simulink library "Kitchen_Lib"  (R2023a)
settings: Solver=VariableStepAuto  StartTime=0.0  StopTime=10.0  RelTol=1e-3  EnableMultiTasking=on
undefined symbols (not defined in the file): Kitc_BusTyp_P, Kitc_BusTypSkyr_C, Kitc_ColrLedColrls_C, Kitc_ColrLedGrn_C, Kitc_ColrLedRed_C, Kitc_ColrLedYlw_C, Kitc_StDgnWtrTank_C, Kitc_StElecPlugScktOffByClmp50_P, Kitc_StsDlyBlink_C, Kitc_StsErrBlink_C, Kitc_StsFctAcvn_P, Kitc_StsInfoBlink_C, Kitc_StsKitchnOffAutoIgOff_P, Kitc_StsKitchnOffBySwt_P, Kitc_StsKitchnOffDoorLockd_P, Kitc_StsKitchnOffIgOff_P, Kitc_StsKitchnOffUv_P, Kitc_StsKitchnOnBySwt_P, Kitc_StsKitchnOnNVM_P, Kitc_StsLedOff_C, Kitc_StsLedOn_C, Kitc_StsLrgCnsAcv_P, Kitc_StTrfrAnSwtInstd_P, Kitc_StTrfrSwtInstd_P, Kitc_TiKitcRefgtrOffDly_P, Kitc_ULowrThdBat_C, Kitc_UUpprThdBat_C, Kitc_ValFalse_C, Kitc_ValPwmFreq2_C, Kitc_ValPwmFreq_C, Kitc_ValTrue_C
libraries: MAN_Library x50, E2E_Lib x3
(part 5 of 13)

== system Kitchen_Lib/Kitchen/100ms/Kitchn/Subsystem1/Subsystem9/BOOLEAN_TO_UINT8_Signals ==
  BOOLEAN_TO_UINT8_SignalIn : Inport
  Constant : Constant  Value=uint8(0)
  Constant1 : Constant  Value=uint8(1)
  Constant2 : Constant  Value=uint8(2)
  Constant3 : Constant  Value=uint8(3)
  Data Type Conversion : DataTypeConversion  OutDataTypeStr=uint8  SaturateOnIntegerOverflow=off  RndMeth=Floor
  Relational Operator{,1..3} (4 alike) : RelationalOperator  Operator===  OutDataTypeStr=boolean  InputSameDT=off
  SignalOff : Outport
  Signal|On : Outport  Port=2
  Error : Outport  Port=3
  NotInstalled_NotAvailable : Outport  Port=4
  wires:
  Relational Operator3/1 -> NotInstalled_NotAvailable/1
  Relational Operator2/1 -> Error/1
  Relational Operator1/1 -> Signal|On/1
  Relational Operator/1 -> SignalOff/1
  Data Type Conversion/1 -> Relational Operator/1, Relational Operator2/1, Relational Operator3/1, Relational Operator1/1
  Constant2/1 -> Relational Operator2/2
  Constant/1 -> Relational Operator/2
  BOOLEAN_TO_UINT8_SignalIn/1 -> Data Type Conversion/1
  Constant3/1 -> Relational Operator3/2
  Constant1/1 -> Relational Operator1/2

== system Kitchen_Lib/Kitchen/100ms/Kitchn/Subsystem1/Subsystem16/001_KitchnCtl/001_HostessSideButton ==
  GW_SpdGrtr3 : Inport
  DBF_StsDoor1Open : Inport  Port=2
  Kitc_StKitcHostsSideSwtUpprPart : Inport  Port=3
  Kitc_StKitcHostsSideSwtBotmPart : Inport  Port=4
  "GW_ModeExbn " : Inport  Port=5
  "GW_StUvTopPrio " : Inport  Port=6
  Kitchn_On : Inport  Port=7
  001_HostessSideTopButton : Subsystem
  002_HostessSideBottomButton : Subsystem
  Logical Operator18 : Logic  AllPortsSameDT=off  OutDataTypeStr=boolean
  Logical Operator19 : Logic  Operator=NOT  Inputs=4  AllPortsSameDT=off  OutDataTypeStr=boolean
  HostsSideTopBtnErr : Outport
  HostsSideBotmBtnErr : Outport  Port=2
  HostsSideTopBtn_ON : Outport  Port=3
  HostsSideBotmBtn_OFF : Outport  Port=4
  wires:
  Logical Operator18/1 -> 001_HostessSideTopButton/2(SwtLock), 002_HostessSideBottomButton/4(SwtLock)
  002_HostessSideBottomButton/1(HostessSideBottomButtonErr) -> HostsSideBotmBtnErr/1
  "GW_ModeExbn "/1 -> 001_HostessSideTopButton/3("GW_ModeExbn "), 002_HostessSideBottomButton/2("GW_ModeExbn ")
  001_HostessSideTopButton/2(HostessSideBottomButton_ON) -> HostsSideTopBtn_ON/1
  GW_SpdGrtr3/1 -> Logical Operator19/1
  002_HostessSideBottomButton/2(HostessSideBottomButton_OFF) -> HostsSideBotmBtn_OFF/1
  Kitchn_On/1 -> 002_HostessSideBottomButton/1(Kitchn_On), 001_HostessSideTopButton/5(Kitchn_On)
  Logical Operator19/1 -> Logical Operator18/1
  Kitc_StKitcHostsSideSwtUpprPart/1 -> 001_HostessSideTopButton/1(Kitc_StKitcHostsSideSwtUpprPart)
  001_HostessSideTopButton/1(HostessSideTopButtonErr) -> HostsSideTopBtnErr/1
  DBF_StsDoor1Open/1 -> Logical Operator18/2
  "GW_StUvTopPrio "/1 -> 001_HostessSideTopButton/4("GW_StUvTopPrio ")
  Kitc_StKitcHostsSideSwtBotmPart/1 -> 002_HostessSideBottomButton/3(Kitc_StKitcHostsSideSwtBotmPart)

== system Kitchen_Lib/Kitchen/100ms/Kitchn/Subsystem1/Subsystem16/001_KitchnCtl/002_FlipFlop ==
  Kitc_StsHostsCallAcv : Inport
  Kitc_StKitcSwtUpprPart : Inport  Port=2
  HostsSideTopBtn_ON : Inport  Port=3
  HostsSideBotmBtn_OFF : Inport  Port=4
  Kitc_StKitcSwtBotmPart : Inport  Port=5
  CLS_StDoorLockdOutd : Inport  Port=6
  "GW_StStrtNew " : Inport  Port=7
  "GW_ModeExbn " : Inport  Port=8
  "GW_StUvTopPrio " : Inport  Port=9
  GW_StClmp15 : Inport  Port=10
  ABat_StAddlBatInstd : Inport  Port=11
  GW_StEngRung : Inport  Port=12
  "GW_Ubat " : Inport  Port=13
  "GW_StClmp50Off3Sec " : Inport  Port=14
  Kitc_StDemoBd : Inport  Port=15
  Kitc_TdOff : Inport  Port=16
  KSW-KitchenControl : Subsystem
  KitchenEnable : Subsystem
  LrgCns : Outport
  Kitc_WarnLrgCns : Outport  Port=2
  Kitchn_On : Outport  Port=3
  Kitc_StsKitcAcv : Outport  Port=4
  Kitchn_HostsCallOn : Outport  Port=5
  Kitc_StLrgCns : Outport  Port=6
  Kitc_StSmlCns : Outport  Port=7
  Kitc_StWtrPump : Outport  Port=8
  Kitc_StBuzRe : Outport  Port=9
  Kitc_StKitcLi : Outport  Port=10
  Kitc_StsPwmFreq : Outport  Port=11
  wires:
  Kitc_StKitcSwtUpprPart/1 -> KitchenEnable/1(Kitc_StKitcSwtUpprPart)
  HostsSideTopBtn_ON/1 -> KitchenEnable/2(HostsSideTopBtn_ON)
  HostsSideBotmBtn_OFF/1 -> KitchenEnable/3(HostsSideBotmBtn_OFF)
  Kitc_StKitcSwtBotmPart/1 -> KitchenEnable/4(Kitc_StKitcSwtBotmPart)
  CLS_StDoorLockdOutd/1 -> [CLS_StDoorLockdOutd]
  "GW_StStrtNew "/1 -> KitchenEnable/6("GW_StStrtNew ")
  "GW_ModeExbn "/1 -> [GW_ModeExbn]
  "GW_StUvTopPrio "/1 -> [GW_StUvTopPrio]
  GW_StClmp15/1 -> [GW_StClmp15]
  Kitc_StDemoBd/1 -> KitchenEnable/10(Kitc_StDemoBd)
  Kitc_TdOff/1 -> KitchenEnable/11(Kitc_TdOff)
  KitchenEnable/1(Kitchn_On) -> KSW-KitchenControl/10(Kitchn_On), Kitchn_On/1
  ABat_StAddlBatInstd/1 -> KSW-KitchenControl/1(ABat_StAddlBatInstd)
  GW_StEngRung/1 -> KSW-KitchenControl/2(GW_StEngRung)
  "GW_Ubat "/1 -> KSW-KitchenControl/3("GW_Ubat ")
  "GW_StClmp50Off3Sec "/1 -> KSW-KitchenControl/4("GW_StClmp50Off3Sec ")
  Kitc_StsHostsCallAcv/1 -> KSW-KitchenControl/6(Kitc_StsHostsCallAcv)
  KSW-KitchenControl/1(LrgCns) -> LrgCns/1
  KSW-KitchenControl/8(Kitc_StBuzRe) -> Kitc_StBuzRe/1
  KSW-KitchenControl/5(Kitc_StLrgCns) -> Kitc_StLrgCns/1
  KSW-KitchenControl/4(Kitchn_HostsCallOn) -> Kitchn_HostsCallOn/1
  KSW-KitchenControl/3(Kitc_StsKitcAcv) -> Kitc_StsKitcAcv/1
  KSW-KitchenControl/2(Kitc_WarnLrgCns) -> Kitc_WarnLrgCns/1
  KSW-KitchenControl/6(Kitc_StSmlCns) -> Kitc_StSmlCns/1
  KSW-KitchenControl/9(Kitc_StKitcLi) -> Kitc_StKitcLi/1
  KSW-KitchenControl/7(Kitc_StWtrPump) -> Kitc_StWtrPump/1
  [CLS_StDoorLockdOutd] -> KitchenEnable/5(CLS_StDoorLockdOutd)
  [GW_ModeExbn] -> KitchenEnable/7("GW_ModeExbn ")
  [GW_StUvTopPrio] -> KitchenEnable/8("GW_StUvTopPrio ")
  [GW_StClmp15] -> KitchenEnable/9(GW_StClmp15)
  [GW_ModeExbn] -> KSW-KitchenControl/7("GW_ModeExbn ")
  [GW_StUvTopPrio] -> KSW-KitchenControl/8("GW_StUvTopPrio ")
  [GW_StClmp15] -> KSW-KitchenControl/9(GW_StClmp15)
  [CLS_StDoorLockdOutd] -> KSW-KitchenControl/5(CLS_StDoorLockdOutd)
  KSW-KitchenControl/10(Kitc_StsPwmFreq) -> Kitc_StsPwmFreq/1

== system Kitchen_Lib/Kitchen/100ms/Kitchn/Subsystem1/Subsystem16/001_KitchnCtl/003_KitchenDriver ==
  note: 3_78_R_Kueche_treiber_83258850004
  Kitc_StHostsCallBlink : Inport
  Kitc_StHostsCallBlinkUpprDeck : Inport  Port=2
  Kitc_StsWtrTankEmpty : Inport  Port=3
  "GW_StrtLock " : Inport  Port=4
  "GW_StClmp15On3Sec " : Inport  Port=5
  Diagnostic : Subsystem
  Logical Operator1 : Logic  Operator=OR  AllPortsSameDT=off  OutDataTypeStr=boolean
  Kitc_StHostsCall : Outport
  wires:
  Logical Operator1/1 -> Kitc_StHostsCall/1
  Kitc_StHostsCallBlink/1 -> Logical Operator1/1
  Kitc_StHostsCallBlinkUpprDeck/1 -> Logical Operator1/2
  Kitc_StsWtrTankEmpty/1 -> Diagnostic/1(Kitc_StsWtrTankEmpty)
  "GW_StrtLock "/1 -> Diagnostic/2("GW_StrtLock ")
  "GW_StClmp15On3Sec "/1 -> Diagnostic/3("GW_StClmp15On3Sec ")

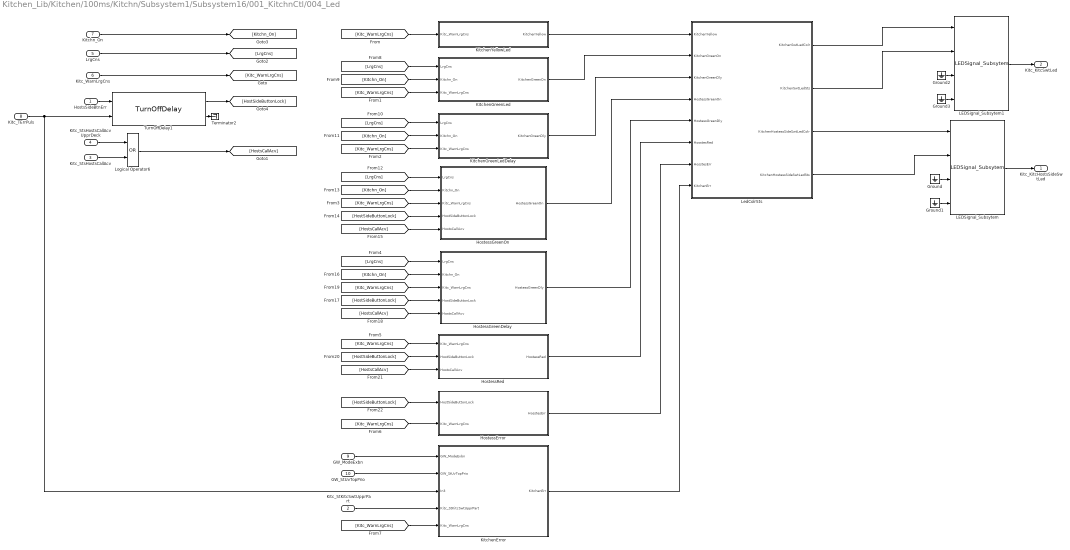
== system Kitchen_Lib/Kitchen/100ms/Kitchn/Subsystem1/Subsystem16/001_KitchnCtl/004_Led ==
  HostsSideBtnErr : Inport
  Kitc_StKitcSwtUpprPart : Inport  Port=2
  Kitc_StsHostsCallAcv : Inport  Port=3
  Kitc_StsHostsCallAcvUpprDeck : Inport  Port=4
  LrgCns : Inport  Port=5
  Kitc_WarnLrgCns : Inport  Port=6
  Kitchn_On : Inport  Port=7
  Kitc_TErrPuls : Inport  Port=8
  "GW_ModeExbn " : Inport  Port=9
  "GW_StUvTopPrio " : Inport  Port=10
  Ground{,1..3} (4 alike) : Ground
  HostessError : Subsystem
  HostessGreenDelay : Subsystem
  HostessGreenOn : Subsystem
  HostessRed : Subsystem
  KitchenError : Subsystem
  KitchenGreenLed : Subsystem
  KitchenGreenLedDelay : Subsystem
  KitchenYellowLed : Subsystem
  LEDSignal_Subsytem : E2E_Lib/LEDSignal_Subsytem
  LEDSignal_Subsytem1 : E2E_Lib/LEDSignal_Subsytem
  LedColrSts : Subsystem
  Logical Operator6 : Logic  Operator=OR  AllPortsSameDT=off  OutDataTypeStr=boolean
  Terminator2 : Terminator
  TurnOffDelay1 : MAN_Library/TurnOffDelay  CycleTime=Cycle Time: 10 Ms
  Kitc_KitcHostsSideSwtLed : Outport
  Kitc_KitcSwtLed : Outport  Port=2
  wires:
  LedColrSts/1(KitchenSwtLedColr) -> LEDSignal_Subsytem1/1
  LedColrSts/2(KitchenSwtLedSts) -> LEDSignal_Subsytem1/2
  Kitc_WarnLrgCns/1 -> [Kitc_WarnLrgCns]
  KitchenYellowLed/1(KitchenYellow) -> LedColrSts/1(KitchenYellow)
  KitchenGreenLed/1(KitchenGreenOn) -> LedColrSts/2(KitchenGreenOn)
  KitchenGreenLedDelay/1(KitchenGreenDly) -> LedColrSts/3(KitchenGreenDly)
  HostessGreenOn/1(HostessGreenOn) -> LedColrSts/4(HostessGreenOn)
  HostessGreenDelay/1(HostessGreenDly) -> LedColrSts/5(HostessGreenDly)
  HostessRed/1(HostessRed) -> LedColrSts/6(HosstesRed)
  HostessError/1(HosstesErr) -> LedColrSts/7(HosstesErr)
  "GW_ModeExbn "/1 -> KitchenError/1("GW_ModeExbn ")
  "GW_StUvTopPrio "/1 -> KitchenError/2("GW_StUvTopPrio ")
  Kitc_StKitcSwtUpprPart/1 -> KitchenError/4(Kitc_StKitcSwtUpprPart)
  KitchenError/1(KitchenErr) -> LedColrSts/8(KitchenErr)
  TurnOffDelay1/1 -> [HostSideButtonLock]
  TurnOffDelay1/2 -> Terminator2/1
  HostsSideBtnErr/1 -> TurnOffDelay1/1
  Kitc_StsHostsCallAcv/1 -> Logical Operator6/2
  Kitc_StsHostsCallAcvUpprDeck/1 -> Logical Operator6/1
  Kitc_TErrPuls/1 -> KitchenError/3(In3), TurnOffDelay1/2
  Logical Operator6/1 -> [HostsCallAcv]
  LrgCns/1 -> [LrgCns]
  Kitchn_On/1 -> [Kitchn_On]
  [Kitc_WarnLrgCns] -> KitchenYellowLed/1(Kitc_WarnLrgCns)
  [Kitc_WarnLrgCns] -> KitchenGreenLed/3(Kitc_WarnLrgCns)
  [Kitc_WarnLrgCns] -> KitchenGreenLedDelay/3(Kitc_WarnLrgCns)
  [Kitc_WarnLrgCns] -> HostessGreenOn/3(Kitc_WarnLrgCns)
  [Kitc_WarnLrgCns] -> HostessRed/1(Kitc_WarnLrgCns)
  [Kitc_WarnLrgCns] -> HostessError/2(Kitc_WarnLrgCns)
  [Kitc_WarnLrgCns] -> KitchenError/5(Kitc_WarnLrgCns)
  [LrgCns] -> KitchenGreenLed/1(LrgCns)
  [Kitchn_On] -> KitchenGreenLed/2(Kitchn_On)
  [Kitchn_On] -> KitchenGreenLedDelay/2(Kitchn_On)
  [LrgCns] -> KitchenGreenLedDelay/1(LrgCns)
  [Kitchn_On] -> HostessGreenOn/2(Kitchn_On)
  [LrgCns] -> HostessGreenOn/1(LrgCns)
  [HostSideButtonLock] -> HostessGreenOn/4(HostSideButtonLock)
  [HostsCallAcv] -> HostessGreenOn/5(HostsCallAcv)
  [Kitc_WarnLrgCns] -> HostessGreenDelay/3(Kitc_WarnLrgCns)
  [LrgCns] -> HostessGreenDelay/1(LrgCns)
  [Kitchn_On] -> HostessGreenDelay/2(Kitchn_On)
  [HostSideButtonLock] -> HostessGreenDelay/4(HostSideButtonLock)
  [HostsCallAcv] -> HostessGreenDelay/5(HostsCallAcv)
  [HostSideButtonLock] -> HostessRed/2(HostSideButtonLock)
  [HostsCallAcv] -> HostessRed/3(HostsCallAcv)
  [HostSideButtonLock] -> HostessError/1(HostSideButtonLock)
  Ground/1 -> LEDSignal_Subsytem/3
  Ground1/1 -> LEDSignal_Subsytem/4
  LEDSignal_Subsytem/1 -> Kitc_KitcHostsSideSwtLed/1
  LedColrSts/3(KitchenHostessSideSwtLedColr) -> LEDSignal_Subsytem/1
  LedColrSts/4(KitchenHostessSideSwtLedSts) -> LEDSignal_Subsytem/2
  LEDSignal_Subsytem1/1 -> Kitc_KitcSwtLed/1
  Ground2/1 -> LEDSignal_Subsytem1/3
  Ground3/1 -> LEDSignal_Subsytem1/4

== system Kitchen_Lib/Kitchen/100ms/Kitchn/Subsystem1/Subsystem16/004_Trfr/001_AutomaticControlKitchenRelease ==
  GW_StClmp15 : Inport
  "GW_StUvNormPrio " : Inport  Port=2
  ABat_StAddlBatInstd : Inport  Port=3
  GW_StEngRung : Inport  Port=4
  Kitc_StsKitcAcv : Inport  Port=5
  Logical Operator : Logic  Operator=NOT  AllPortsSameDT=off  OutDataTypeStr=boolean
  Logical Operator3 : Logic  Inputs=4  AllPortsSameDT=off  OutDataTypeStr=boolean
  Logical Operator4 : Logic  Operator=OR  AllPortsSameDT=off  OutDataTypeStr=boolean
  Kitchen : Outport
  wires:
  "GW_StUvNormPrio "/1 -> Logical Operator/1
  GW_StEngRung/1 -> Logical Operator4/2
  ABat_StAddlBatInstd/1 -> Logical Operator4/1
  Logical Operator4/1 -> Logical Operator3/2
  GW_StClmp15/1 -> Logical Operator3/3
  Logical Operator3/1 -> Kitchen/1
  Logical Operator/1 -> Logical Operator3/4
  Kitc_StsKitcAcv/1 -> Logical Operator3/1

== system Kitchen_Lib/Kitchen/100ms/Kitchn/Subsystem1/Subsystem16/004_Trfr/002_FlipFlop ==
  TrfrSwt : Inport
  Kitc_StTrfrSwtUpprPart : Inport  Port=2
  Kitc_StTrfrSwtTopBtn : Inport  Port=3
  Kitc_StTrfrSwtLowrPart : Inport  Port=4
  Kitc_StTrfrBotmBtm : Inport  Port=5
  "GW_StStrtNew " : Inport  Port=6
  Kitc_StTrfrWoutNewStrt : Inport  Port=7
  GW_StEngRung : Inport  Port=8
  ABat_StAddlBatInstd : Inport  Port=9
  GW_StClmp15 : Inport  Port=10
  "GW_StUvNormPrio " : Inport  Port=11
  KSW-Nvm : Subsystem
  Kitc_StsTurnOnByBtnNv : DataStoreRead  DataStoreName=Kitc_StsTurnOnByBtnNv  IndexOptions=Index vector (dialog)  Indices=1  OutputSizes=1
  Logical Operator5 : Logic  Operator=OR  Inputs=4  AllPortsSameDT=off  OutDataTypeStr=boolean
  NvM_ActiveOnlyForFirstCycle : MAN_Library/NvM_ActiveOnlyForFirstCycle
  StateChangePulse : MAN_Library/StateChangePulse
  TurnOffByButton : Subsystem
  TurnOffConditions : Subsystem
  TurnOnByButton : Subsystem
  TurnOnNvm : Subsystem
  Unit Delay : UnitDelay  SampleTime=-1  HasFrameUpgradeWarning=on
  Fnc_On : Outport
  wires:
  StateChangePulse/1 -> Unit Delay/1, Fnc_On/1
  Logical Operator5/1 -> StateChangePulse/1
  Unit Delay/1 -> [Fnc_ON]
  "GW_StStrtNew "/1 -> KSW-Nvm/3("GW_StStrtNew ")
  [TurnOff] -> KSW-Nvm/2(TurnOff)
  Kitc_StTrfrWoutNewStrt/1 -> KSW-Nvm/4(Kitc_StTrfrWoutNewStrt)
  [TurnOn] -> KSW-Nvm/1(TurnOn)
  ABat_StAddlBatInstd/1 -> [ABat_StAddlBatInstd]
  GW_StEngRung/1 -> [GW_StEngRung]
  GW_StClmp15/1 -> [GW_StClmp15]
  "GW_StUvNormPrio "/1 -> [GW_StUvNormPrio]
  Kitc_StsTurnOnByBtnNv/1 -> NvM_ActiveOnlyForFirstCycle/1
  TurnOnByButton/1(TurnOn) -> Logical Operator5/1, [TurnOn]
  Kitc_StTrfrSwtUpprPart/1 -> TurnOnByButton/1(Kitc_StTrfrSwtUpprPart)
  Kitc_StTrfrSwtTopBtn/1 -> TurnOnByButton/2(Kitc_StTrfrSwtTopBtn)
  TurnOffByButton/1(TurnOff) -> [TurnOff], Logical Operator5/2
  Kitc_StTrfrSwtLowrPart/1 -> TurnOffByButton/1(Kitc_StTrfrSwtLowrPart)
  Kitc_StTrfrBotmBtm/1 -> TurnOffByButton/2(Kitc_StTrfrBotmBtm)
  TurnOffConditions/1(CdnOff) -> Logical Operator5/3
  TrfrSwt/1 -> TurnOnNvm/1(TrfrSwt)
  TurnOnNvm/1(TurnOnNvm) -> Logical Operator5/4
  [Fnc_ON] -> TurnOnByButton/7(Fnc_ON)
  [Fnc_ON] -> TurnOffByButton/3(Fnc_ON)
  [GW_StUvNormPrio] -> TurnOnByButton/6("GW_StUvNormPrio ")
  [GW_StClmp15] -> TurnOnByButton/5(GW_StClmp15)
  [ABat_StAddlBatInstd] -> TurnOnByButton/4(ABat_StAddlBatInstd)
  [GW_StEngRung] -> TurnOnByButton/3(GW_StEngRung)
  [GW_StEngRung] -> TurnOffConditions/1(GW_StEngRung)
  [ABat_StAddlBatInstd] -> TurnOffConditions/2(ABat_StAddlBatInstd)
  [GW_StClmp15] -> TurnOffConditions/3(GW_StClmp15)
  [GW_StUvNormPrio] -> TurnOffConditions/4("GW_StUvNormPrio ")
  [Fnc_ON] -> TurnOffConditions/5(Fnc_ON)
  [GW_StEngRung] -> TurnOnNvm/3(GW_StEngRung)
  [ABat_StAddlBatInstd] -> TurnOnNvm/4(ABat_StAddlBatInstd)
  [GW_StClmp15] -> TurnOnNvm/5(GW_StClmp15)
  [GW_StUvNormPrio] -> TurnOnNvm/7(GW_StUvNormPrio)
  [Fnc_ON] -> TurnOnNvm/6(Fnc_ON)
  NvM_ActiveOnlyForFirstCycle/1 -> TurnOnNvm/2(Kitc_StsTurnOnByBtnNv)

== system Kitchen_Lib/Kitchen/100ms/Kitchn/Subsystem1/Subsystem16/004_Trfr/003_TrfrSwtLed ==
  Fnc_On : Inport
  Constant12 : Constant  Value=Kitc_ColrLedColrls_C
  Constant13 : Constant  Value=Kitc_ColrLedYlw_C
  Constant4 : Constant  Value=Kitc_StsLedOff_C
  Constant5 : Constant  Value=Kitc_StsLedOn_C
  Multiport Switch1 : MultiPortSwitch  DataPortOrder=Zero-based contiguous  Inputs=2  zeroidx=on  SaturateOnIntegerOverflow=off  InputSameDT=off
  Multiport Switch2 : MultiPortSwitch  DataPortOrder=Zero-based contiguous  Inputs=2  zeroidx=on  SaturateOnIntegerOverflow=off  InputSameDT=off
  Kitc_ColrTrfrSwtLed : Outport
  Kitc_StsTrfrSwtLed : Outport  Port=2
  wires:
  Constant5/1 -> Multiport Switch2/3
  Constant4/1 -> Multiport Switch2/2
  Constant12/1 -> Multiport Switch1/2
  Constant13/1 -> Multiport Switch1/3
  Multiport Switch1/1 -> Kitc_ColrTrfrSwtLed/1
  Multiport Switch2/1 -> Kitc_StsTrfrSwtLed/1
  Fnc_On/1 -> Multiport Switch1/1, Multiport Switch2/1

== system Kitchen_Lib/Kitchen/100ms/Kitchn/Subsystem1/Subsystem16/004_Trfr/PushPull ==
  In1 : Inport
  Constant : Constant  Value=Kitc_ValFalse_C
  "Constant1                                                                 " : MAN_Library/TimeConstant  hours=0  minutes=0  seconds=0  miliseconds=50
  Terminator : Terminator
  TurnOnDelay : MAN_Library/TurnOnDelay  CycleTime=Cycle Time: 10 Ms
  HS : Outport
  LS : Outport  Port=2
  wires:
  In1/1 -> TurnOnDelay/1
  Constant/1 -> LS/1
  TurnOnDelay/1 -> HS/1
  "Constant1                                                                 "/1 -> TurnOnDelay/2
  TurnOnDelay/2 -> Terminator/1

== system Kitchen_Lib/Kitchen/100ms/Kitchn/Subsystem1/Subsystem19/003_TrfrSwtLed/LEDSignal_Subsytem ==
  note: Output Led SignalValue
      | Led Signal Blink Info
      | Led Signal Color Info
      |
      | 0
      | Off
      |
      | 1
      | 200/800
      |
      | green
      |
      | 2
      | 250/250
      |
      | green
      |
      | 3
      | 800/200
      |
      | green
      |
      | 4
      | 100%
      |
      | green
      |
      | 5
      | 200/800
      | yellow
      |
      | 6
      | 250/250
      | yellow
      |
      | 7
      | 800/200
      |
      | yellow
      |
      | 8
      | 100%
      |
      | yellow
      |
      | 9
      | 200/800
      | red
      |
      | 10
      | 250/250
      | red
      |
      | 11
      | 800/200
      |
      | red
      |
      | 12
      | 100%
      |
      | red
      |
      | 14
      | Error
      |
      | 15
      | NA
  note: Off
  note: Blink Info
      | Value
      |
      | Led off
      | 0
      |
      | Led on
      | 1
      |
      | Led 500ms on 500ms off
      | 2
      |
      | Led 250ms on 250ms off
      | 3
      |
      | Led200ms on 800ms off
      | 4
      |
      | Led 800ms on 200ms off
      | 5
  note: Led Info
      | Value
      |
      | Yellow
      | 2
      |
      | Green
      | 3
      |
      | Red
      | 1
  note: 800/200
  note: 500/500
  note: 200/800
  note: 250/250
  note: 100
  note: 800/200
  note: 500/500
  note: 200/800
  note: 250/250
  note: 100
  note: 800/200
  note: 500/500
  note: 200/800
  note: 250/250
  note: 100
  note: Off
  note: Off
  Color : Inport
  Status : Inport  Port=2
  Error : Inport  Port=3
  NA : Inport  Port=4
  Constant{1..5,56,61,66} (8 alike) : Constant  Value=uint8(0)
  Constant55 : Constant  Value=uint8(4)
  Constant57 : Constant  Value=uint8(2)
  Constant58 : Constant  Value=uint8(1)
  Constant59 : Constant  Value=uint8(3)
  Constant60 : Constant  Value=uint8(8)
  Constant62 : Constant  Value=uint8(6)
  Constant63 : Constant  Value=uint8(5)
  Constant64 : Constant  Value=uint8(7)
  Constant65 : Constant  Value=uint8(12)
  Constant67 : Constant  Value=uint8(10)
  Constant68 : Constant  Value=uint8(9)
  Constant69 : Constant  Value=uint8(11)
  Constant70 : Constant  Value=uint8(14)
  Constant71 : Constant  Value=uint8(16)
  Ground : Ground
  Ground1 : Ground
  Ground2 : Ground
  Multiport Switch17 : MultiPortSwitch  DataPortOrder=Zero-based contiguous  Inputs=6  DataPortForDefault=Additional data port  zeroidx=on  SaturateOnIntegerOverflow=off  InputSameDT=off
  Multiport Switch23 : MultiPortSwitch  DataPortOrder=Zero-based contiguous  Inputs=4  DataPortForDefault=Additional data port  DiagnosticForDefault=None  zeroidx=on  SaturateOnIntegerOverflow=off  InputSameDT=off
  Multiport Switch24 : MultiPortSwitch  DataPortOrder=Zero-based contiguous  Inputs=6  DataPortForDefault=Additional data port  zeroidx=on  SaturateOnIntegerOverflow=off  InputSameDT=off
  Multiport Switch25 : MultiPortSwitch  DataPortOrder=Zero-based contiguous  Inputs=6  DataPortForDefault=Additional data port  zeroidx=on  SaturateOnIntegerOverflow=off  InputSameDT=off
  Multiport Switch26 : MultiPortSwitch  DataPortOrder=Zero-based contiguous  Inputs=2  zeroidx=on  SaturateOnIntegerOverflow=off  InputSameDT=off
  Multiport Switch27 : MultiPortSwitch  DataPortOrder=Zero-based contiguous  Inputs=2  zeroidx=on  SaturateOnIntegerOverflow=off  InputSameDT=off
  Led : Outport
  wires:
  Status/1 -> Multiport Switch25/1, Multiport Switch24/1, Multiport Switch17/1
  Multiport Switch17/1 -> Multiport Switch23/5
  Multiport Switch24/1 -> Multiport Switch23/4
  Multiport Switch25/1 -> Multiport Switch23/3
  Constant1/1 -> Multiport Switch23/6
  Constant5/1 -> Multiport Switch23/2
  Constant57/1 -> Multiport Switch17/5
  Constant64/1 -> Multiport Switch24/7
  Ground1/1 -> Multiport Switch24/4
  Constant60/1 -> Multiport Switch24/3
  Constant62/1 -> Multiport Switch24/5
  Constant63/1 -> Multiport Switch24/6
  Constant61/1 -> Multiport Switch24/2
  Multiport Switch26/1 -> Multiport Switch27/2
  Multiport Switch23/1 -> Multiport Switch26/2
  Error/1 -> Multiport Switch26/1
  Constant69/1 -> Multiport Switch25/7
  Constant67/1 -> Multiport Switch25/5
  Ground2/1 -> Multiport Switch25/4
  Constant66/1 -> Multiport Switch25/2
  Constant68/1 -> Multiport Switch25/6
  Constant65/1 -> Multiport Switch25/3
  Constant70/1 -> Multiport Switch26/3
  Constant71/1 -> Multiport Switch27/3
  Color/1 -> Multiport Switch23/1
  Constant58/1 -> Multiport Switch17/6
  Constant55/1 -> Multiport Switch17/3
  NA/1 -> Multiport Switch27/1
  Constant56/1 -> Multiport Switch17/2
  Ground/1 -> Multiport Switch17/4
  Constant59/1 -> Multiport Switch17/7
  Multiport Switch27/1 -> Led/1
  Constant2/1 -> Multiport Switch24/8
  Constant3/1 -> Multiport Switch17/8
  Constant4/1 -> Multiport Switch25/8

== system Kitchen_Lib/Kitchen/100ms/Kitchn/Subsystem1/Subsystem19/Cluster_Message/Subsystem2 ==
  Not_Released : Subsystem
  Released : Subsystem
  Subsystem : Subsystem
  Subsystem1 : Subsystem
  Out1 : Outport
  Out2 : Outport  Port=2
  wires:
  Not_Released/1(Kitc_StClusterNotReleased) -> Out1/1
  Not_Released/2(Kitc_StClusterLowBtNotReleased) -> Out2/1
  [GW_StUvTopPrio] -> Subsystem1/2(GW_StUvTopPrio)
  [GW_StClmp15] -> Subsystem1/4(GW_StClmp15)
  Subsystem1/1(NotReleasedCondition) -> Not_Released/Enable
  [Kitc_StKitcSwtUpprPart] -> Not_Released/1(Released_Button)
  Subsystem/1(Out1) -> Released/Enable
  [Kitc_StKitcSwtUpprPart] -> Subsystem1/3(Kitc_StKitcSwtUpprPart)
  [GW_StUvTopPrio] -> Not_Released/2(GW_StUvTopPrio)
  [SleepMode] -> Subsystem1/5(SleepMode)
  [Kitc_StKitcSwtUpprPart] -> Released/1(Released_Button)
  [GW_StUvTopPrio] -> Subsystem/1(GW_StUvTopPrio)
  [Kitc_StKitcSwtUpprPart] -> Subsystem/2(Kitc_StKitcSwtUpprPart)
  Released/1(Kitc_StClusterKitchnReleased) -> Subsystem1/1(Kitc_StClusterKitchnReleased), Not_Released/3(Kitc_StClusterKitchnReleased)

== system Kitchen_Lib/Kitchen/100ms/Kitchn/Subsystem1/Subsystem19/KSW_Battery/BatteryVoltageUnder22700mV ==
  Kitchn_On : Inport
  EngOrAddlBat : Inport  Port=2
  "GW_Ubat " : Inport  Port=3
  Constant : Constant  Value=Kitc_StsLrgCnsAcv_P
  Constant2 : Constant  Value=Kitc_ULowrThdBat_C
  Data Store Read : DataStoreRead  DataStoreName=Kitc_StsLrgCnsAcvNv  IndexOptions=Index vector (dialog)  Indices=1  OutputSizes=1
  Data Type Conversion : DataTypeConversion  OutDataTypeStr=boolean  SaturateOnIntegerOverflow=off  RndMeth=Floor
  Logical Operator1 : Logic  Operator=NOT  Inputs=4  AllPortsSameDT=off  OutDataTypeStr=boolean
  Logical Operator2 : Logic  Inputs=4  AllPortsSameDT=off  OutDataTypeStr=boolean
  Relational Operator1 : RelationalOperator  Operator=<=  OutDataTypeStr=boolean  InputSameDT=off
  Switch : Switch  Criteria=u2 ~= 0  SaturateOnIntegerOverflow=off  InputSameDT=off
  BatUUnder22700mV : Outport
  wires:
  Data Type Conversion/1 -> Switch/2
  Constant/1 -> Switch/3
  Data Store Read/1 -> Switch/1, Data Type Conversion/1
  Logical Operator2/1 -> BatUUnder22700mV/1
  EngOrAddlBat/1 -> Logical Operator1/1
  "GW_Ubat "/1 -> Relational Operator1/1
  Constant2/1 -> Relational Operator1/2
  Relational Operator1/1 -> Logical Operator2/4
  Logical Operator1/1 -> Logical Operator2/1
  Switch/1 -> Logical Operator2/3
  Kitchn_On/1 -> Logical Operator2/2

== system Kitchen_Lib/Kitchen/100ms/Kitchn/Subsystem1/Subsystem19/KSW_Battery/BatteryVoltageUnder23V ==
  GW_Ubat : Inport
  EngOrAddlBat : Inport  Port=2
  Kitchn_On : Inport  Port=3
  Kitc_StsHostsCallAcv : Inport  Port=4
  Constant : Constant  Value=Kitc_StsLrgCnsAcv_P
  Constant1 : Constant  Value=Kitc_UUpprThdBat_C
  "Constant3  " : Subsystem  AncestorBlock=MAN_Library/TimeConstant  mask{hours=0, minutes=0, seconds=10, miliseconds=0}
      mask prompts: hours "Hour"
      mask DialogControl TimeConstant Prompt: Time Constant
      mask Display:
      | timeDraw = 'Time#';
      | if( hours == 0 && minutes == 0 && seconds == 0 && miliseconds == 0)
      |     timeDraw = strcat(timeDraw,'0secs'),
      | else
      |     if( hours ~= 0)
      |         timeDraw = strcat(timeDraw,num2str(hours),'hours');
      |     end
      |     if( minutes ~= 0)
      |         timeDraw = strcat(timeDraw,num2str(minutes),'min');
      |     end
      |     if( seconds ~= 0)
      |         timeDraw = strcat(timeDraw,num2str(seconds),'sec');
      |     end
      |     if( miliseconds ~= 0)
      |         timeDraw = strcat(timeDraw,num2str(miliseconds),'ms');
      |     end
      | end
      | fprintf(timeDraw);
  "Constant4  " : Subsystem  AncestorBlock=MAN_Library/TimeConstant  mask{hours=0, minutes=10, seconds=0, miliseconds=0}
      mask prompts: hours "Hour"
      mask DialogControl TimeConstant Prompt: Time Constant
      mask Display:
      | timeDraw = 'Time#';
      | if( hours == 0 && minutes == 0 && seconds == 0 && miliseconds == 0)
      |     timeDraw = strcat(timeDraw,'0secs'),
      | else
      |     if( hours ~= 0)
      |         timeDraw = strcat(timeDraw,num2str(hours),'hours');
      |     end
      |     if( minutes ~= 0)
      |         timeDraw = strcat(timeDraw,num2str(minutes),'min');
      |     end
      |     if( seconds ~= 0)
      |         timeDraw = strcat(timeDraw,num2str(seconds),'sec');
      |     end
      |     if( miliseconds ~= 0)
      |         timeDraw = strcat(timeDraw,num2str(miliseconds),'ms');
      |     end
      | end
      | fprintf(timeDraw);
  "Constant6  " : Subsystem  AncestorBlock=MAN_Library/TimeConstant  mask{hours=0, minutes=0, seconds=0, miliseconds=500}
      mask prompts: hours "Hour"
      mask DialogControl TimeConstant Prompt: Time Constant
      mask Display:
      | timeDraw = 'Time#';
      | if( hours == 0 && minutes == 0 && seconds == 0 && miliseconds == 0)
      |     timeDraw = strcat(timeDraw,'0secs'),
      | else
      |     if( hours ~= 0)
      |         timeDraw = strcat(timeDraw,num2str(hours),'hours');
      |     end
      |     if( minutes ~= 0)
      |         timeDraw = strcat(timeDraw,num2str(minutes),'min');
      |     end
      |     if( seconds ~= 0)
      |         timeDraw = strcat(timeDraw,num2str(seconds),'sec');
      |     end
      |     if( miliseconds ~= 0)
      |         timeDraw = strcat(timeDraw,num2str(miliseconds),'ms');
      |     end
      | end
      | fprintf(timeDraw);
  Data Store Read : DataStoreRead  DataStoreName=Kitc_StsLrgCnsAcvNv  IndexOptions=Index vector (dialog)  Indices=1  OutputSizes=1
  Data Type Conversion : DataTypeConversion  OutDataTypeStr=boolean  SaturateOnIntegerOverflow=off  RndMeth=Floor
  Logical Operator15 : Logic  Operator=OR  AllPortsSameDT=off  OutDataTypeStr=boolean
  Logical Operator16 : Logic  Operator=NOT  Inputs=4  AllPortsSameDT=off  OutDataTypeStr=boolean
  Logical Operator3 : Logic  Inputs=4  AllPortsSameDT=off  OutDataTypeStr=boolean
  Logical Operator4 : Logic  Operator=NOT  Inputs=4  AllPortsSameDT=off  OutDataTypeStr=boolean
  Relational Operator : RelationalOperator  Operator=<=  OutDataTypeStr=boolean  InputSameDT=off
  Switch : Switch  Criteria=u2 ~= 0  SaturateOnIntegerOverflow=off  InputSameDT=off
  Terminator : Terminator
  Terminator1 : Terminator
  Terminator2 : Terminator
  TimePulse : Subsystem  AncestorBlock=MAN_Library/TimePulse  mask(Time Pulse){CycleTime=Cycle Time: 10 Ms}
      mask prompts: CycleTime "Select the Cycle Time:"
      mask help:
      | This is a PULSE GENERATOR producing a pulse, if there is a positive-going edge at input IN. The length of the pulse which should be generated is defined by input PT. After the occurrence of the positive edge output Q is set to HIGH for the period of time defined in PT. Output ET counts the time - beginning with the occurrence of the positive edge - until the value set at PT has been reached. The value in ET is kept as long as the input IN has the state of HIGH.
      |
      | IN : Timer starting bit
      | PT : Preset time of timer
      | Q  : Time pulse flag
      | ET : Current value of timer
      mask TypeOptions CycleTime: Cycle Time: 1 Ms | Cycle Time: 10 Ms | Cycle Time: 100 Ms | Cycle Time: 1000 Ms
      mask Display:
      | disp('{\bf\fontsize{18}Time Pulse}', 'texmode','on');
      | 
      | port_label('input', 1,'IN');
      | port_label('input', 2,'PT');
      | port_label('output',1,'Q');
      | port_label('output',2,'ET');
  TimePulse1 : Subsystem  AncestorBlock=MAN_Library/TimePulse  mask(Time Pulse){CycleTime=Cycle Time: 10 Ms}
      mask prompts: CycleTime "Select the Cycle Time:"
      mask help:
      | This is a PULSE GENERATOR producing a pulse, if there is a positive-going edge at input IN. The length of the pulse which should be generated is defined by input PT. After the occurrence of the positive edge output Q is set to HIGH for the period of time defined in PT. Output ET counts the time - beginning with the occurrence of the positive edge - until the value set at PT has been reached. The value in ET is kept as long as the input IN has the state of HIGH.
      |
      | IN : Timer starting bit
      | PT : Preset time of timer
      | Q  : Time pulse flag
      | ET : Current value of timer
      mask TypeOptions CycleTime: Cycle Time: 1 Ms | Cycle Time: 10 Ms | Cycle Time: 100 Ms | Cycle Time: 1000 Ms
      mask Display:
      | disp('{\bf\fontsize{18}Time Pulse}', 'texmode','on');
      | 
      | port_label('input', 1,'IN');
      | port_label('input', 2,'PT');
      | port_label('output',1,'Q');
      | port_label('output',2,'ET');
  TurnOffDelay : Subsystem  AncestorBlock=MAN_Library/TurnOffDelay  mask(Turn Off Delay){CycleTime=Cycle Time: 10 Ms}
      mask prompts: CycleTime "Select the Cycle Time:"
      mask help:
      | This is an EDGE DELAY where the turning-off edge is delayed. The delay period is entered at input PT. The output Q is reset after turning off input IN, only after the delay period is over. Output ET counts the time - beginning with the occurrence of the negative edge - until the value set at PT has been reached. The output ET shows the expired time since turning input IN off until the input state of IN is put through to output Q.
      |
      | IN : Timer starting bit
      | PT : Preset time of timer
      | Q  : Time pulse flag
      | ET : Current value of timer
      mask TypeOptions CycleTime: Cycle Time: 1 Ms | Cycle Time: 10 Ms | Cycle Time: 100 Ms | Cycle Time: 1000 Ms
      mask Display:
      | disp('{\bf\fontsize{18}Turn Off Delay}', 'texmode','on');
      | 
      | port_label('input', 1,'IN');
      | port_label('input', 2,'PT');
      | port_label('output',1,'Q');
      | port_label('output',2,'ET');
  LrgCnsOff : Outport
  Kitc_WarnLrgCns : Outport  Port=2
  Kitc_StBuzRe : Outport  Port=3
  wires:
  Data Type Conversion/1 -> Switch/2
  Constant/1 -> Switch/3
  Data Store Read/1 -> Switch/1, Data Type Conversion/1
  Switch/1 -> Logical Operator3/3
  Constant1/1 -> Relational Operator/2
  Relational Operator/1 -> Logical Operator3/4
  Kitchn_On/1 -> Logical Operator3/2
  Logical Operator16/1 -> Logical Operator3/1
  EngOrAddlBat/1 -> Logical Operator16/1
  GW_Ubat/1 -> Relational Operator/1
  "Constant3  "/1(time) -> TimePulse/2(TimePulseDuration)
  TimePulse/1(TimePulseFlag) -> Kitc_WarnLrgCns/1, Logical Operator15/1
  "Constant4  "/1(time) -> TurnOffDelay/2(TurnOffDelayThreshold)
  Logical Operator4/1 -> TurnOffDelay/1(TurnOffDelayEnable)
  TurnOffDelay/1(TurnOffDelayFlag) -> LrgCnsOff/1
  Kitc_StsHostsCallAcv/1 -> TimePulse1/1(TimePulseEnable)
  Logical Operator15/1 -> Kitc_StBuzRe/1
  "Constant6  "/1(time) -> TimePulse1/2(TimePulseDuration)
  TimePulse1/1(TimePulseFlag) -> Logical Operator15/2
  TurnOffDelay/2(TurnOffDelayExpiredTime) -> Terminator/1
  TimePulse/2(TimePulseExpiredTime) -> Terminator1/1
  TimePulse1/2(TimePulseExpiredTime) -> Terminator2/1
  Logical Operator3/1 -> Logical Operator4/1, TimePulse/1(TimePulseEnable)

== system Kitchen_Lib/Kitchen/100ms/Kitchn/Subsystem1/Subsystem19/KSW_Battery/KitchenActivation ==
  note: Large Comsp
  "GW_StClmp50Off3Sec " : Inport
  "GW_StUvTopPrio " : Inport  Port=2
  "GW_ModeExbn " : Inport  Port=3
  CLS_StDoorLockdOutd : Inport  Port=4
  BatUUnder22.7V : Inport  Port=5
  LrgCnsOff : Inport  Port=6
  Kitchn_On : Inport  Port=7
  GW_StClmp15 : Inport  Port=8
  EngOrAddlBat : Inport  Port=9
  Constant : Constant  Value=Kitc_StsLrgCnsAcv_P
  Data Store Read : DataStoreRead  DataStoreName=Kitc_StsLrgCnsAcvNv  IndexOptions=Index vector (dialog)  Indices=1  OutputSizes=1
  Data Type Conversion : DataTypeConversion  OutDataTypeStr=boolean  SaturateOnIntegerOverflow=off  RndMeth=Floor
  Logical Operator{1,9..12} (5 alike) : Logic  Operator=NOT  Inputs=4  AllPortsSameDT=off  OutDataTypeStr=boolean
  Logical Operator13 : Logic  Operator=OR  AllPortsSameDT=off  OutDataTypeStr=boolean
  Logical Operator5 : Logic  Operator=OR  AllPortsSameDT=off  OutDataTypeStr=boolean
  Logical Operator6 : Logic  Inputs=3  AllPortsSameDT=off  OutDataTypeStr=boolean
  Logical Operator7 : Logic  Inputs=9  AllPortsSameDT=off  OutDataTypeStr=boolean
  Switch : Switch  Criteria=u2 ~= 0  SaturateOnIntegerOverflow=off  InputSameDT=off
  Terminator : Terminator
  wires:
  Data Type Conversion/1 -> Switch/2
  Constant/1 -> Switch/3
  Data Store Read/1 -> Switch/1, Data Type Conversion/1
  Logical Operator13/1 -> Terminator/1
  Logical Operator6/1 -> Logical Operator5/2
  Logical Operator5/1 -> Logical Operator13/1
  Logical Operator11/1 -> Logical Operator7/1
  Logical Operator9/1 -> Logical Operator7/2
  "GW_StUvTopPrio "/1 -> Logical Operator9/1
  Logical Operator12/1 -> Logical Operator7/4
  Switch/1 -> Logical Operator7/5
  Logical Operator7/1 -> Logical Operator5/1
  "GW_ModeExbn "/1 -> Logical Operator10/1
  Logical Operator10/1 -> Logical Operator7/3
  CLS_StDoorLockdOutd/1 -> Logical Operator12/1
  "GW_StClmp50Off3Sec "/1 -> Logical Operator11/1
  GW_StClmp15/1 -> Logical Operator7/8, Logical Operator6/2
  BatUUnder22.7V/1 -> Logical Operator1/1
  Kitchn_On/1 -> Logical Operator6/1, [Kitchn_On], Logical Operator7/9
  LrgCnsOff/1 -> Logical Operator7/7
  EngOrAddlBat/1 -> Logical Operator6/3
  Logical Operator1/1 -> Logical Operator7/6
  [Kitchn_On] -> Logical Operator13/2

== system Kitchen_Lib/Kitchen/100ms/Kitchn/Subsystem1/Subsystem19/KitchenEnable/001_HostessSideButton ==
  note: TBoE
  note: TBuE
  Kitc_StKitcHostsSideSwtBotmPart : Inport
  Kitc_StKitcHostsSideSwtUpprPart : Inport  Port=2
  GW_SpdGrtr3 : Inport  Port=3
  DBF_StsDoor1Open : Inport  Port=4
  Kitchn_On : Inport  Port=5
  "GW_StUvTopPrio " : Inport  Port=6
  "GW_ModeExbn " : Inport  Port=7
  001_HostessSideTopButton : Subsystem
  002_HostessSideBottomButton : Subsystem
  Logical Operator18 : Logic  AllPortsSameDT=off  OutDataTypeStr=boolean
  Logical Operator19 : Logic  Operator=NOT  Inputs=4  AllPortsSameDT=off  OutDataTypeStr=boolean
  Logical Operator7 : Logic  Operator=OR  AllPortsSameDT=off  OutDataTypeStr=boolean
  HostsSideBotmBtn_OFF : Outport
  HostsSideBtnErr : Outport  Port=2
  wires:
  002_HostessSideBottomButton/1(HostessSideBottomButtonErr) -> Logical Operator7/2
  Kitc_StKitcHostsSideSwtBotmPart/1 -> 002_HostessSideBottomButton/3(Kitc_StKitcHostsSideSwtBotmPart)
  "GW_StUvTopPrio "/1 -> 001_HostessSideTopButton/4("GW_StUvTopPrio ")
  DBF_StsDoor1Open/1 -> Logical Operator18/2
  Kitc_StKitcHostsSideSwtUpprPart/1 -> 001_HostessSideTopButton/1(Kitc_StKitcHostsSideSwtUpprPart)
  Logical Operator19/1 -> Logical Operator18/1
  Kitchn_On/1 -> 002_HostessSideBottomButton/1(Kitchn_On)
  002_HostessSideBottomButton/2(HostessSideBottomButton_OFF) -> HostsSideBotmBtn_OFF/1
  GW_SpdGrtr3/1 -> Logical Operator19/1
  "GW_ModeExbn "/1 -> 002_HostessSideBottomButton/2("GW_ModeExbn "), 001_HostessSideTopButton/3("GW_ModeExbn ")
  Logical Operator18/1 -> 002_HostessSideBottomButton/4(SwtLock), 001_HostessSideTopButton/2(SwtLock)
  001_HostessSideTopButton/1(HostessSideTopButtonErr) -> Logical Operator7/1
  Logical Operator7/1 -> HostsSideBtnErr/1

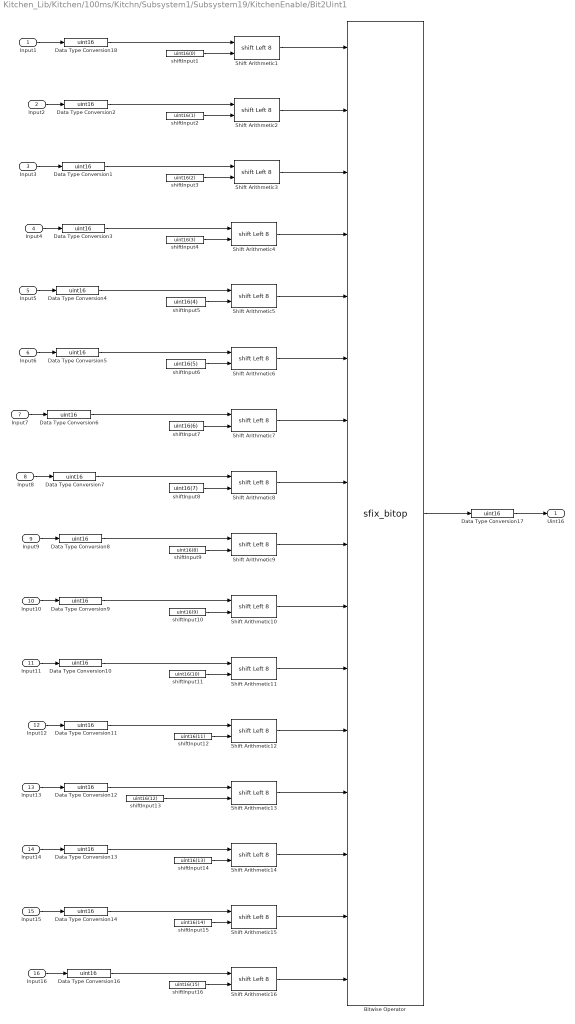
== system Kitchen_Lib/Kitchen/100ms/Kitchn/Subsystem1/Subsystem19/KitchenEnable/Bit2Uint1 ==
  Input1 : Inport
  Input2 : Inport  Port=2
  Input3 : Inport  Port=3
  Input4 : Inport  Port=4
  Input5 : Inport  Port=5
  Input6 : Inport  Port=6
  Input7 : Inport  Port=7
  Input8 : Inport  Port=8
  Input9 : Inport  Port=9
  Input10 : Inport  Port=10
  Input11 : Inport  Port=11
  Input12 : Inport  Port=12
  Input13 : Inport  Port=13
  Input14 : Inport  Port=14
  Input15 : Inport  Port=15
  Input16 : Inport  Port=16
  Bitwise Operator : S-Function  AncestorBlock=|  FunctionName=sfix_bitop  Parameters=UseBitMask,NumInputPorts,BitMask,BitMaskRealWorld,logicop  SFunctionDeploymentMode=off  EnableBusSupport=off  mask(Bitwise Operator){logicop=OR, UseBitMask=off, NumInputPorts=16, BitMask=bin2dec('11011001'), BitMaskRealWorld=Stored Integer}
      | simulink/Logic and Bit
      | Operations/Bitwise
      | Operator
      mask prompts: logicop "Simulink:masks:Operator_MP"; UseBitMask "Simulink:masks:UseBitMask_MP"; NumInputPorts "Simulink:masks:NumberOfInputPorts_MP"; BitMask "Simulink:masks:BitMask_MP"; BitMaskRealWorld "Simulink:masks:TreatMaskAs_MP"
      mask help: Simulink:masks:BitwiseOperator_MD
      mask init:
      | str = '';
      | if UseBitMask
      |   [m,n] = size(BitMask);
      |   if ischar(BitMask)
      |     len = m;
      |     n = 1;
      |   else
      |     len = m * n;
      |   end
      |   internalBitMask = zeros(m,n);
      |   if isnumeric(BitMask)
      |     if ~isreal(BitMask)
      |       error(DAStudio.message('Simulink:blocks:BitMaskNotComplex'));
      |     end
      |     for i=1:len,
      |       internalBitMask(i) = BitMask(i);
      |     end
      |   elseif ischar(BitMask)
      |     for i=1:m,
      |       internalBitMask(i) = hex2dec(BitMask(i,:));
      |     end
      |   elseif iscell(BitMask)
      |     for i=1:len,
      |       if isnumeric( BitMask{i} )
      |         internalBitMask(i) = BitMask{i};
      |       elseif ischar( BitMask{i} )
      |         internalBitMask(i) = hex2dec(BitMask{i});
      |       else
      |         errordlg(['Data type is not supported at cell item ', num2str(i) ]);
      |       end
      |     end
      |   end
      |   BitMask = internalBitMask;
      |   for i=1:len
      |     if BitMask(i) > (2^52)-1
      |       error(DAStudio.message('Simulink:blocks:BitMaskWordLengthTooLarge')); 
      |     end
      |   end 
      |   if len == 1
      |      if BitMaskRealWorld == 1 || BitMask(1) < 0
      |        str=num2str(BitMask(1));
      |      else
      |        str=['0x',dec2hex(floor(BitMask(1)))];
      |      end
      |   else
      |      str='Masks';
      |   end
      | else
      |   BitMask = 0;
      |   str='';
      | end
      mask TypeOptions logicop: Simulink:masks:AND | Simulink:masks:OR | Simulink:masks:NAND | Simulink:masks:NOR | Simulink:masks:XOR | Simulink:masks:NOT
      mask Callback logicop: fixptdialog(gcbh)
      mask Callback UseBitMask: fixptdialog(gcbh)
      mask TypeOptions BitMaskRealWorld: Simulink:masks:RealWorldValue | Simulink:masks:StoredInteger
      mask Display: fprintf(['Bitwise\n',logicop,'\n',str])
  Data Type Conversion{1..14,16..18} (17 alike) : DataTypeConversion  OutDataTypeStr=uint16  SaturateOnIntegerOverflow=off  RndMeth=Floor
  Shift Arithmetic{1..16} (16 alike) : ArithShift  BitShiftNumberSource=Input port  BitShiftNumber=8  BitShiftDirection=Left
      settings: InputPortMap=u0,p1
  shiftInput1 : Constant  Value=uint16(0)  SampleTime=-1
  shiftInput10 : Constant  Value=uint16(9)  SampleTime=-1
  shiftInput11 : Constant  Value=uint16(10)  SampleTime=-1
  shiftInput12 : Constant  Value=uint16(11)  SampleTime=-1
  shiftInput13 : Constant  Value=uint16(12)  SampleTime=-1
  shiftInput14 : Constant  Value=uint16(13)  SampleTime=-1
  shiftInput15 : Constant  Value=uint16(14)  SampleTime=-1
  shiftInput16 : Constant  Value=uint16(15)  SampleTime=-1
  shiftInput2 : Constant  Value=uint16(1)  SampleTime=-1
  shiftInput3 : Constant  Value=uint16(2)  SampleTime=-1
  shiftInput4 : Constant  Value=uint16(3)  SampleTime=-1
  shiftInput5 : Constant  Value=uint16(4)  SampleTime=-1
  shiftInput6 : Constant  Value=uint16(5)  SampleTime=-1
  shiftInput7 : Constant  Value=uint16(6)  SampleTime=-1
  shiftInput8 : Constant  Value=uint16(7)  SampleTime=-1
  shiftInput9 : Constant  Value=uint16(8)  SampleTime=-1
  Uint16 : Outport
  wires:
  Shift Arithmetic16/1 -> Bitwise Operator/16
  Shift Arithmetic15/1 -> Bitwise Operator/15
  Shift Arithmetic14/1 -> Bitwise Operator/14
  Shift Arithmetic13/1 -> Bitwise Operator/13
  Shift Arithmetic12/1 -> Bitwise Operator/12
  Shift Arithmetic11/1 -> Bitwise Operator/11
  Shift Arithmetic10/1 -> Bitwise Operator/10
  Shift Arithmetic9/1 -> Bitwise Operator/9
  Data Type Conversion16/1 -> Shift Arithmetic16/1
  shiftInput16/1 -> Shift Arithmetic16/2
  Input16/1 -> Data Type Conversion16/1
  Data Type Conversion14/1 -> Shift Arithmetic15/1
  shiftInput15/1 -> Shift Arithmetic15/2
  Input15/1 -> Data Type Conversion14/1
  Data Type Conversion13/1 -> Shift Arithmetic14/1
  shiftInput14/1 -> Shift Arithmetic14/2
  Input14/1 -> Data Type Conversion13/1
  Data Type Conversion12/1 -> Shift Arithmetic13/1
  shiftInput13/1 -> Shift Arithmetic13/2
  Input13/1 -> Data Type Conversion12/1
  Data Type Conversion11/1 -> Shift Arithmetic12/1
  shiftInput12/1 -> Shift Arithmetic12/2
  Input12/1 -> Data Type Conversion11/1
  Data Type Conversion10/1 -> Shift Arithmetic11/1
  shiftInput11/1 -> Shift Arithmetic11/2
  Input11/1 -> Data Type Conversion10/1
  Data Type Conversion9/1 -> Shift Arithmetic10/1
  shiftInput10/1 -> Shift Arithmetic10/2
  Input10/1 -> Data Type Conversion9/1
  Data Type Conversion8/1 -> Shift Arithmetic9/1
  shiftInput9/1 -> Shift Arithmetic9/2
  Input9/1 -> Data Type Conversion8/1
  Data Type Conversion7/1 -> Shift Arithmetic8/1
  Data Type Conversion6/1 -> Shift Arithmetic7/1
  Data Type Conversion5/1 -> Shift Arithmetic6/1
  Data Type Conversion4/1 -> Shift Arithmetic5/1
  Data Type Conversion3/1 -> Shift Arithmetic4/1
  Data Type Conversion1/1 -> Shift Arithmetic3/1
  Data Type Conversion2/1 -> Shift Arithmetic2/1
  Data Type Conversion18/1 -> Shift Arithmetic1/1
  shiftInput1/1 -> Shift Arithmetic1/2
  shiftInput2/1 -> Shift Arithmetic2/2
  Input1/1 -> Data Type Conversion18/1
  Input2/1 -> Data Type Conversion2/1
  shiftInput3/1 -> Shift Arithmetic3/2
  Input3/1 -> Data Type Conversion1/1
  shiftInput4/1 -> Shift Arithmetic4/2
  Input4/1 -> Data Type Conversion3/1
  shiftInput5/1 -> Shift Arithmetic5/2
  Input5/1 -> Data Type Conversion4/1
  shiftInput6/1 -> Shift Arithmetic6/2
  Input6/1 -> Data Type Conversion5/1
  shiftInput7/1 -> Shift Arithmetic7/2
  Input7/1 -> Data Type Conversion6/1
  shiftInput8/1 -> Shift Arithmetic8/2
  Input8/1 -> Data Type Conversion7/1
  Shift Arithmetic1/1 -> Bitwise Operator/1
  Shift Arithmetic2/1 -> Bitwise Operator/2
  Shift Arithmetic3/1 -> Bitwise Operator/3
  Shift Arithmetic4/1 -> Bitwise Operator/4
  Shift Arithmetic5/1 -> Bitwise Operator/5
  Shift Arithmetic6/1 -> Bitwise Operator/6
  Shift Arithmetic7/1 -> Bitwise Operator/7
  Shift Arithmetic8/1 -> Bitwise Operator/8
  Bitwise Operator/1 -> Data Type Conversion17/1
  Data Type Conversion17/1 -> Uint16/1

== system Kitchen_Lib/Kitchen/100ms/Kitchn/Subsystem1/Subsystem19/KitchenEnable/KitchenOffAutomaticIgnitionOff ==
  Kitc_StDemoBd : Inport
  Kitc_TdOff : Inport  Port=2
  GW_StClmp15 : Inport  Port=3
  Kitchen_On : Inport  Port=4
  "Constant4           " : Subsystem  AncestorBlock=MAN_Library/TimeConstant  mask{hours=0, minutes=0, seconds=10, miliseconds=0}
      mask prompts: hours "Hour"
      mask DialogControl TimeConstant Prompt: Time Constant
      mask Display:
      | timeDraw = 'Time#';
      | if( hours == 0 && minutes == 0 && seconds == 0 && miliseconds == 0)
      |     timeDraw = strcat(timeDraw,'0secs'),
      | else
      |     if( hours ~= 0)
      |         timeDraw = strcat(timeDraw,num2str(hours),'hours');
      |     end
      |     if( minutes ~= 0)
      |         timeDraw = strcat(timeDraw,num2str(minutes),'min');
      |     end
      |     if( seconds ~= 0)
      |         timeDraw = strcat(timeDraw,num2str(seconds),'sec');
      |     end
      |     if( miliseconds ~= 0)
      |         timeDraw = strcat(timeDraw,num2str(miliseconds),'ms');
      |     end
      | end
      | fprintf(timeDraw);
  Logical Operator36 : Logic  AllPortsSameDT=off  OutDataTypeStr=boolean
  Logical Operator37 : Logic  Operator=NOT  Inputs=4  AllPortsSameDT=off  OutDataTypeStr=boolean
  Multiport Switch2 : MultiPortSwitch  DataPortOrder=Zero-based contiguous  Inputs=2  zeroidx=on  SaturateOnIntegerOverflow=off  InputSameDT=off
  RisingEdgeDetection2 : Subsystem  AncestorBlock=MAN_Library/RisingEdgeDetection
  Terminator : Terminator
  TurnOnDelay : Subsystem  AncestorBlock=MAN_Library/TurnOnDelay  mask(Turn On Delay){CycleTime=Cycle Time: 10 Ms}
      mask prompts: CycleTime "Select the Cycle Time:"
      mask help:
      | This is an EDGE DELAY where the turning-on edge is delayed. The delay period is entered at input PT. Output Q is set on TRUE after turning on input IN, only after the delay period is over. Output ET counts the time - beginning with the occurrence of the positive edge - until the value set at PT has been reached. The output ET shows the expired time since turning input IN on until the input state of IN is put through to output Q.
      |
      | IN : Timer starting bit
      | PT : Preset time of timer
      | Q  : Time up flag
      | ET : Current value of timer
      mask TypeOptions CycleTime: Cycle Time: 1 Ms | Cycle Time: 10 Ms | Cycle Time: 100 Ms | Cycle Time: 1000 Ms
      mask Display:
      | disp('{\bf\fontsize{18}Turn On Delay}', 'texmode','on');
      | 
      | port_label('input', 1,'IN');
      | port_label('input', 2,'PT');
      | port_label('output',1,'Q');
      | port_label('output',2,'ET');
  "KitchnOffAutoIgOff " : Outport
  wires:
  TurnOnDelay/1(TurnOnDelayFlag) -> RisingEdgeDetection2/1(CLK)
  RisingEdgeDetection2/1(Q) -> "KitchnOffAutoIgOff "/1
  Multiport Switch2/1 -> TurnOnDelay/2(TurnOnDelayThreshold)
  Logical Operator36/1 -> TurnOnDelay/1(TurnOnDelayEnable)
  Logical Operator37/1 -> Logical Operator36/2
  TurnOnDelay/2(TurnOnDelayExpiredTime) -> Terminator/1
  "Constant4           "/1(time) -> Multiport Switch2/3
  Kitc_StDemoBd/1 -> Multiport Switch2/1
  Kitc_TdOff/1 -> Multiport Switch2/2
  Kitchen_On/1 -> Logical Operator36/1
  GW_StClmp15/1 -> Logical Operator37/1

== system Kitchen_Lib/Kitchen/100ms/Kitchn/Subsystem1/Subsystem19/KitchenEnable/KitchenOffBySwitch ==
  Kitc_StKitcSwtBotmPart : Inport
  "GW_ModeExbn " : Inport  Port=2
  Kitchen_On : Inport  Port=3
  Logical Operator20 : Logic  Inputs=3  AllPortsSameDT=off  OutDataTypeStr=boolean
  Logical Operator22 : Logic  Operator=NOT  Inputs=4  AllPortsSameDT=off  OutDataTypeStr=boolean
  KitchnOffBySwt : Outport
  wires:
  Kitc_StKitcSwtBotmPart/1 -> Logical Operator20/1
  Logical Operator20/1 -> KitchnOffBySwt/1
  Logical Operator22/1 -> Logical Operator20/2
  "GW_ModeExbn "/1 -> Logical Operator22/1
  Kitchen_On/1 -> Logical Operator20/3

== system Kitchen_Lib/Kitchen/100ms/Kitchn/Subsystem1/Subsystem19/KitchenEnable/KitchenOffDoorLocked ==
  CLS_StDoorLockdOutd : Inport
  GW_StClmp15 : Inport  Port=2
  Kitchen_On : Inport  Port=3
  Logical Operator39 : Logic  Inputs=3  AllPortsSameDT=off  OutDataTypeStr=boolean
  Logical Operator40 : Logic  Operator=NOT  Inputs=4  AllPortsSameDT=off  OutDataTypeStr=boolean
  RisingEdgeDetection3 : Subsystem  AncestorBlock=MAN_Library/RisingEdgeDetection
  KitchnOffDoorLockd : Outport
  wires:
  GW_StClmp15/1 -> Logical Operator40/1
  Kitchen_On/1 -> Logical Operator39/3
  Logical Operator39/1 -> KitchnOffDoorLockd/1
  RisingEdgeDetection3/1(Q) -> Logical Operator39/2
  CLS_StDoorLockdOutd/1 -> RisingEdgeDetection3/1(CLK)
  Logical Operator40/1 -> Logical Operator39/1

== system Kitchen_Lib/Kitchen/100ms/Kitchn/Subsystem1/Subsystem19/KitchenEnable/KitchenOffIgnitionOff ==
  GW_StClmp15 : Inport
  Kitchen_On : Inport  Port=2
  FallingEdgeDetection : Subsystem  AncestorBlock=MAN_Library/FallingEdgeDetection
  Logical Operator31 : Logic  AllPortsSameDT=off  OutDataTypeStr=boolean
  KitchnOffIgOff : Outport
  wires:
  Kitchen_On/1 -> Logical Operator31/2
  FallingEdgeDetection/1(Q) -> Logical Operator31/1
  Logical Operator31/1 -> KitchnOffIgOff/1
  GW_StClmp15/1 -> FallingEdgeDetection/1(CLK)

== system Kitchen_Lib/Kitchen/100ms/Kitchn/Subsystem1/Subsystem19/KitchenEnable/KitchenOffUndervoltage ==
  "GW_StUvTopPrio " : Inport
  Kitchen_On : Inport  Port=2
  Logical Operator38 : Logic  AllPortsSameDT=off  OutDataTypeStr=boolean
  RisingEdgeDetection4 : Subsystem  AncestorBlock=MAN_Library/RisingEdgeDetection
  KitchnOffUv : Outport
  wires:
  Logical Operator38/1 -> KitchnOffUv/1
  "GW_StUvTopPrio "/1 -> RisingEdgeDetection4/1(CLK)
  RisingEdgeDetection4/1(Q) -> Logical Operator38/2
  Kitchen_On/1 -> Logical Operator38/1
